simulink model "frf_ex3"  (Simulink 9.0)
settings: Solver=ode1  StartTime=0.0  StopTime=SimTime  FixedStep=Ts  RelTol=1e-3  EnableMultiTasking=on
values from neighbouring files (symbols this model uses):
  Ts = 1/1000    (= 0.001)    [exercise_2.m]
settings Model: Creator=witvoetg  LastModifiedBy=Job
settings DataIOCC: SignalLoggingSaveFormat=ModelDataLogs  SignalLoggingName=sigsOut
settings OptimizationCC: InitFltsAndDblsToZero=on
settings DebuggingCC: SaveWithParameterizedLinksMsg=none  SignalResolutionControl=TryResolveAllWithWarning  MultiTaskDSMMsg=warning  MultiTaskCondExecSysMsg=none  FcnCallInpInsideContextMsg=warning
settings HardwareCC: TargetUnknown=on
settings GRTTargetCC: TargetFcnLib=ansi_tfl_tmw.mat  CombineOutputUpdateFcns=off  GRTInterface=on

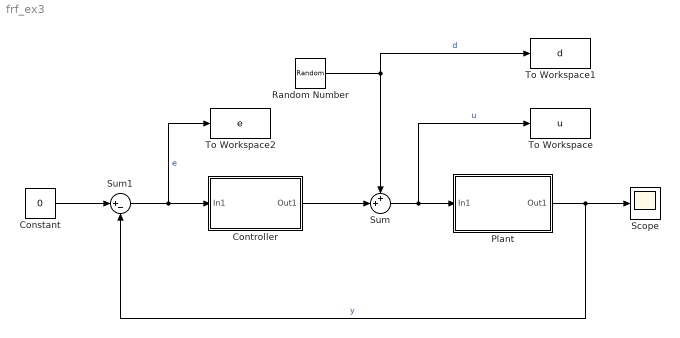
== system frf_ex3 ==
  Constant : Constant  Value=0
  Controller : Subsystem
  Plant : Subsystem
  Random Number : RandomNumber  SampleTime=Ts
  Scope : Scope
  Sum : Sum  Inputs=++|
  Sum1 : Sum  Inputs=|+-  SaturateOnIntegerOverflow=on
  To Workspace : ToWorkspace  VariableName=u  SaveFormat=Timeseries  SampleTime=-1
  To Workspace1 : ToWorkspace  VariableName=d  SaveFormat=Timeseries  SampleTime=-1
  To Workspace2 : ToWorkspace  VariableName=e  SaveFormat=Timeseries  SampleTime=-1
  wires:
  Sum1/1 -> To Workspace2/1, Controller/1(In1)  "e"
  Plant/1(Out1) -> Sum1/2, Scope/1  "y"
  Sum/1 -> To Workspace/1, Plant/1(In1)  "u"
  Controller/1(Out1) -> Sum/2
  Random Number/1 -> To Workspace1/1, Sum/1  "d"
  Constant/1 -> Sum1/1

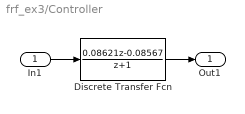
== system frf_ex3/Controller ==
  In1 : Inport
  Discrete Transfer Fcn : DiscreteTransferFcn  Numerator=[0.08621, -0.08567]  Denominator=[1 1]  SampleTime=1/1000
  Out1 : Outport
  wires:
  In1/1 -> Discrete Transfer Fcn/1
  Discrete Transfer Fcn/1 -> Out1/1

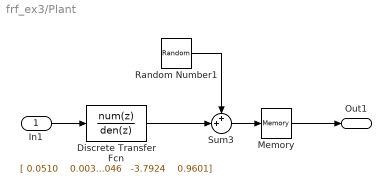
== system frf_ex3/Plant ==
  In1 : Inport
  Discrete Transfer Fcn : DiscreteTransferFcn  Numerator="[ 0.0510    0.0033   -0.0964    0.0012    0.0500]"  Denominator="[1.0000   -3.8723    5.7046   -3.7924    0.9601]"  SampleTime=1/1000
  Memory : Memory
  Random Number1 : RandomNumber  Variance=0.001  Seed=3  SampleTime=0
  Sum3 : Sum  Inputs=++|  SaturateOnIntegerOverflow=on
  Out1 : Outport
  wires:
  Discrete Transfer Fcn/1 -> Sum3/2
  Random Number1/1 -> Sum3/1
  In1/1 -> Discrete Transfer Fcn/1
  Sum3/1 -> Memory/1
  Memory/1 -> Out1/1
